simulink model "Simulator"  (R2023b)
settings: Solver=VariableStepAuto  StartTime=0.0  StopTime=t_sim  RelTol=1e-3
values from neighbouring files (symbols this model uses):
  a_p = 2e-2    (= 0.02)    [Problem_1.m]    (also in Problem_2.m = 0; Problem_3.m = 0.16; Problem_4.m = 0; Problem_5.m)
  a_s = 1e-1    (= 0.1)    [Problem_1.m]    (also in Problem_2.m = 0.01; Problem_3.m = 0.2; Problem_4.m = 0.05; Problem_5.m)
  D_a0 = 5.5e-3    (= 0.0055)    [Problem_1.m]    (also in Problem_2.m = 0.0085; Problem_3.m = 0.0015; Problem_4.m = 0.0025; Problem_5.m)
  D_p0 = 0    [Problem_1.m]    (also in Problem_2.m = 0.003; Problem_3.m; Problem_4.m = 0.0085; Problem_5.m)
  G_a = 0.095    [Problem_1.m]    (also in Problem_2.m = -0.09; Problem_3.m = 0.014; Problem_4.m = 0.006; Problem_5.m = 0.38)
  G_f = 1 / (K_d*G_s)    (= 1)    [Problem_1.m]    (also in Problem_2.m; Problem_3.m; Problem_4.m; Problem_5.m = 0.125)
  G_s = 1    [Problem_1.m]    (also in Problem_2.m; Problem_3.m; Problem_4.m; Problem_5.m = 2)
  K_d = 1    [Problem_1.m]    (also in Problem_2.m; Problem_3.m; Problem_4.m; Problem_5.m = 4)
  w_p = 0.02    [Problem_1.m]    (also in Problem_2.m = 0; Problem_3.m = 0.03; Problem_4.m = 0; Problem_5.m)
  w_s = 40    [Problem_1.m]    (also in Problem_2.m = 50; Problem_3.m = 60; Problem_4.m; Problem_5.m)
libraries: simulink x4, cstblocks x2
settings Model: Creator=vrego  LastModifiedBy=vrego

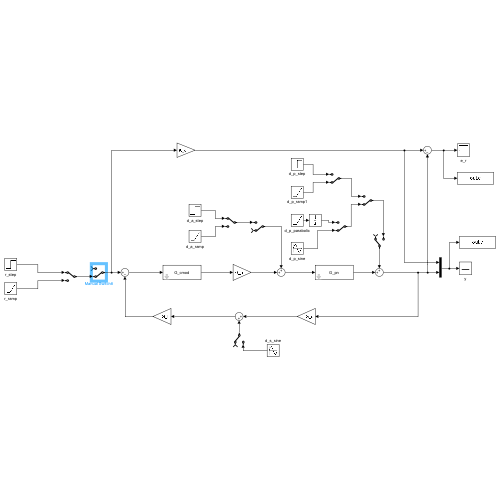
[thumbnail: Simulink's stored preview of the top-level diagram]
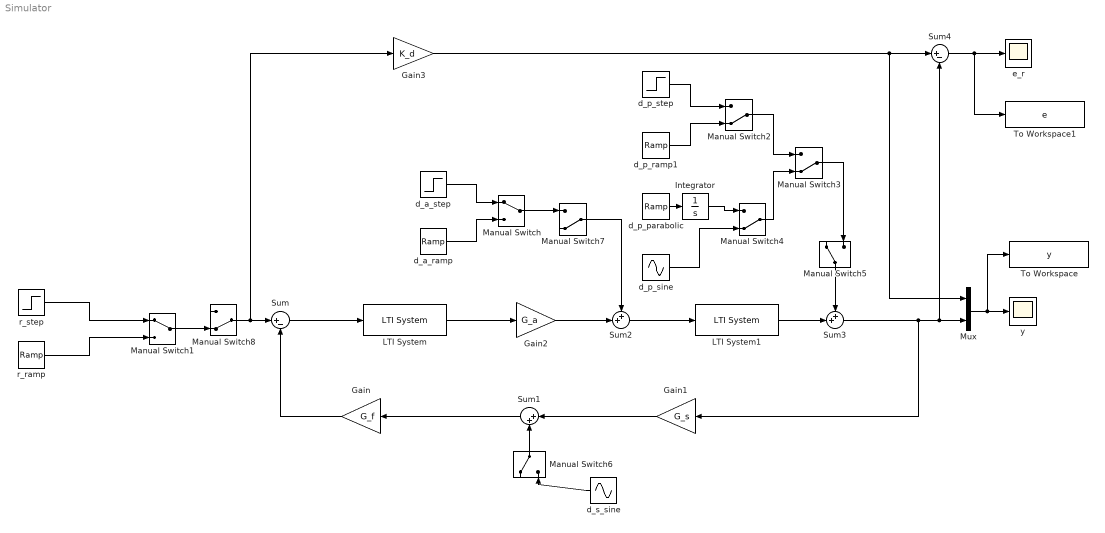
== system Simulator ==
  Gain : Gain  Gain=G_f
  Gain1 : Gain  Gain=G_s
  Gain2 : Gain  Gain=G_a
  Gain3 : Gain  Gain=K_d
  Integrator : Integrator
  LTI System : cstblocks/LTI System  sys=G_cmod  IC=[]  PadeOrder=0
  LTI System1 : cstblocks/LTI System  sys=G_pn  IC=[]  PadeOrder=0
  Manual Switch{,1,5..6} (4 alike) : ManualSwitch
  Manual Switch{2..4,7..8} (5 alike) : ManualSwitch  CurrentSetting=0
  Mux : Mux  Inputs=2
  Sum : Sum  Inputs=|+-
  Sum1 : Sum  Inputs=|++
  Sum2 : Sum  Inputs=++|
  Sum3 : Sum  Inputs=++|
  Sum4 : Sum  Inputs=|+-
  To Workspace : ToWorkspace  VariableName=y  SaveFormat=Timeseries  SampleTime=-1
  To Workspace1 : ToWorkspace  VariableName=e  SaveFormat=Timeseries  SampleTime=-1
  d_a_ramp : simulink/Sources/Ramp  slope=D_a0  start=0  InitialOutput=0
  d_a_step : Step  Time=0  After=D_a0  SampleTime=0
  d_p_parabolic : simulink/Sources/Ramp  slope=2*D_p0  start=0  InitialOutput=0
  d_p_ramp1 : simulink/Sources/Ramp  slope=D_p0  start=0  InitialOutput=0
  d_p_sine : Sin  Amplitude=a_p  Frequency=w_p  SampleTime=0
  d_p_step : Step  Time=0  After=D_p0  SampleTime=0
  d_s_sine : Sin  Amplitude=a_s  Frequency=w_s  SampleTime=0
  e_r : Scope
  r_ramp : simulink/Sources/Ramp  slope=1  start=0  InitialOutput=0
  r_step : Step  Time=0  SampleTime=0
  y : Scope
  wires:
  LTI System/1 -> Gain2/1
  Sum/1 -> LTI System/1
  Gain2/1 -> Sum2/2
  Sum2/1 -> LTI System1/1
  LTI System1/1 -> Sum3/2
  Gain1/1 -> Sum1/1
  Sum1/1 -> Gain/1
  Gain/1 -> Sum/2
  Sum3/1 -> Mux/2, Sum4/2, Gain1/1
  Gain3/1 -> Sum4/1, Mux/1
  Mux/1 -> To Workspace/1, y/1
  Sum4/1 -> To Workspace1/1, e_r/1
  r_step/1 -> Manual Switch1/1
  r_ramp/1 -> Manual Switch1/2
  d_a_step/1 -> Manual Switch/1
  d_a_ramp/1 -> Manual Switch/2
  d_p_step/1 -> Manual Switch2/1
  d_p_ramp1/1 -> Manual Switch2/2
  Manual Switch2/1 -> Manual Switch3/1
  d_p_parabolic/1 -> Integrator/1
  Integrator/1 -> Manual Switch4/1
  d_p_sine/1 -> Manual Switch4/2
  Manual Switch4/1 -> Manual Switch3/2
  Manual Switch3/1 -> Manual Switch5/2
  Manual Switch5/1 -> Sum3/1
  d_s_sine/1 -> Manual Switch6/2
  Manual Switch6/1 -> Sum1/2
  Manual Switch/1 -> Manual Switch7/1
  Manual Switch7/1 -> Sum2/1
  Manual Switch1/1 -> Manual Switch8/2
  Manual Switch8/1 -> Gain3/1, Sum/1
